simulink model "sampleModel1760"  (R2023a)
settings: Solver=VariableStepAuto  StartTime=0.0  StopTime=10.0  RelTol=1e-3
libraries: hdlsllib x6, simulink x5
settings Model: Creator=user1  LastModifiedBy=user1

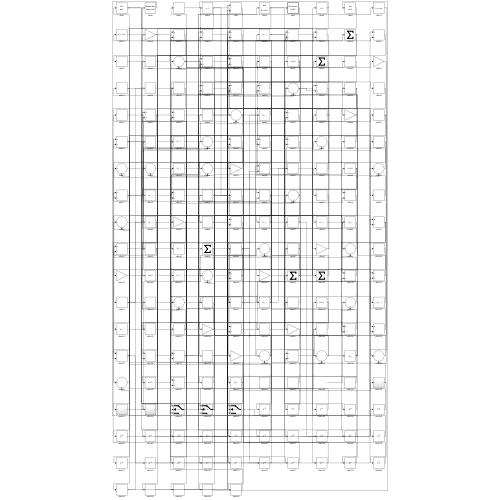
[thumbnail: Simulink's stored preview of the top-level diagram]
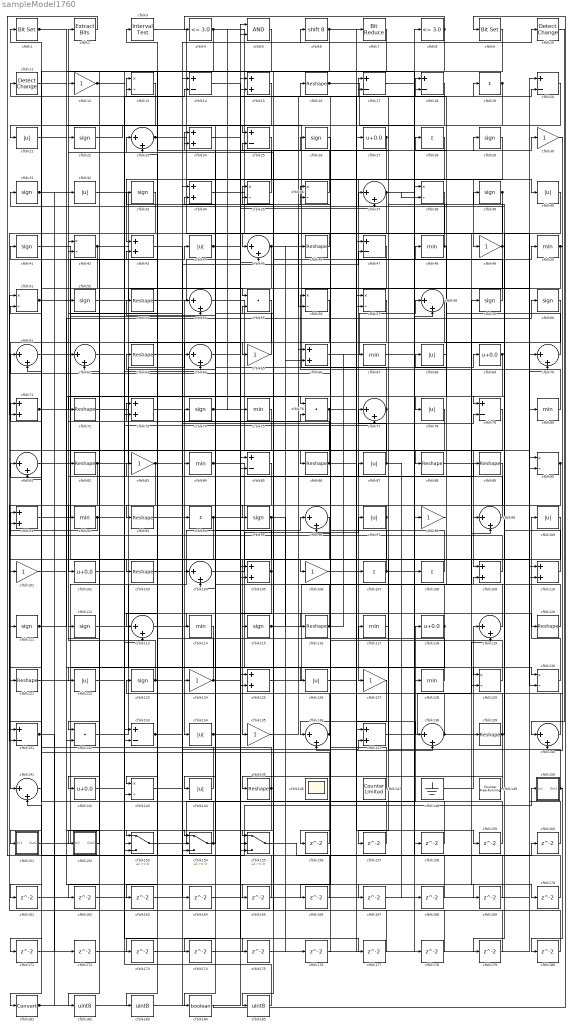
== system sampleModel1760 ==
  cfblk1 : simulink/Logic and Bit Operations/Bit Set  iBit=0
      settings: LibrarySourceBlock=|
      | hdlsllib/Logic and Bit
      | Operations/Bit Set
  cfblk10 : simulink/Logic and Bit Operations/Detect Change  vinit=0  OutDataTypeStr=boolean
      settings: LibrarySourceBlock=|
      | hdlsllib/Logic and Bit
      | Operations/Detect
      | Change
  cfblk{21,32,40,44,68,78,87,97,100,122,126,134,144} (13 alike) : Abs  SaturateOnIntegerOverflow=off
  cfblk{12,30,49,65,83,98,101,106,124,127,135} (11 alike) : Gain
  cfblk{27,69,102,118,142} (5 alike) : Bias  Bias=0.0  SaturateOnIntegerOverflow=off
  cfblk{16,46,53,63,72,82,86,88..89,93,103,116,120..121,139,145} (16 alike) : Reshape
  cfblk{23,37,45,54,58,61..62,64,70,77,81,96,99,104,113,119,136,138,140..141} (20 alike) : Sum  Inputs=|++
  cfblk{15,24,34,43,66,71,73,91,105,109..110,125,137} (13 alike) : Sum
  cfblk{19,28,94,107..108} (5 alike) : Sum  Inputs=+
  cfblk11 : simulink/Logic and Bit Operations/Detect Change  vinit=0  OutDataTypeStr=boolean
      settings: LibrarySourceBlock=|
      | hdlsllib/Logic and Bit
      | Operations/Detect
      | Change
  cfblk{22,26,29,31,33,39,41,52,59..60,74,95,111..112,115,123} (16 alike) : Signum
  cfblk{48,50,67,75,80,84,92,114,117,128} (10 alike) : MinMax
  cfblk{13,35..36,38,42,51,56..57,90,129..130,143} (12 alike) : Product  Inputs=*/  RndMeth=Zero  SaturateOnIntegerOverflow=on
  cfblk{14,17..18,20,25,47,79,85,131,133} (10 alike) : Sum  Inputs=+-
  cfblk132 : DotProduct  OutDataTypeStr=Inherit: Inherit via internal rule
  cfblk146 : Scope
      settings: Floating=on
  cfblk147 : hdlsllib/Sources/Counter Limited  uplimit=7  tsamp=-1
  cfblk148 : Ground
  cfblk149 : hdlsllib/Sources/Counter Free-Running  NumBits=16  tsamp=-1
  cfblk150 : Subsystem
      settings: LibrarySourceBlock=|
      | hdlsllib/Ports &
      | Subsystems/Subsystem
  cfblk151 : Subsystem
      settings: LibrarySourceBlock=|
      | hdlsllib/Ports &
      | Subsystems/Subsystem
  cfblk152 : Subsystem
      settings: LibrarySourceBlock=|
      | hdlsllib/Ports &
      | Subsystems/Subsystem
  cfblk153 : Switch  SaturateOnIntegerOverflow=off  InputSameDT=off
  cfblk154 : Switch  SaturateOnIntegerOverflow=off  InputSameDT=off
  cfblk155 : Switch  SaturateOnIntegerOverflow=off  InputSameDT=off
  cfblk{156..180} (25 alike) : Delay  SampleTime=1
  cfblk181 : DataTypeConversion  SaturateOnIntegerOverflow=off  RndMeth=Floor
  cfblk182 : DataTypeConversion  OutDataTypeStr=uint8  SaturateOnIntegerOverflow=off  RndMeth=Floor
  cfblk183 : DataTypeConversion  OutDataTypeStr=uint8  SaturateOnIntegerOverflow=off  RndMeth=Floor
  cfblk184 : DataTypeConversion  OutDataTypeStr=boolean  SaturateOnIntegerOverflow=off  RndMeth=Floor
  cfblk185 : DataTypeConversion  OutDataTypeStr=uint8  SaturateOnIntegerOverflow=off  RndMeth=Floor
  cfblk2 : simulink/Logic and Bit Operations/Extract Bits  bitsToExtract=Upper half  numBits=8  bitIdxRange=[0 7]  outScalingMode=Preserve fixed-point scaling
      settings: LibrarySourceBlock=|
      | hdlsllib/Logic and Bit
      | Operations/Extract Bits
  cfblk3 : hdlsllib/Logic and Bit Operations/Interval Test  IntervalClosedRight=on  uplimit=0.5  IntervalClosedLeft=on  lowlimit=-0.5  OutDataTypeStr=boolean
  cfblk4 : hdlsllib/Logic and Bit Operations/Compare To Constant  relop=<=  const=3.0  OutDataTypeStr=boolean
  cfblk5 : Logic  AllPortsSameDT=off  OutDataTypeStr=boolean
  cfblk55 : DotProduct  OutDataTypeStr=Inherit: Inherit via internal rule
  cfblk6 : ArithShift  BitShiftNumber=8
  cfblk7 : hdlsllib/Logic and Bit Operations/Bit Reduce  mode=AND
  cfblk76 : DotProduct  OutDataTypeStr=Inherit: Inherit via internal rule
  cfblk8 : hdlsllib/Logic and Bit Operations/Compare To Constant  relop=<=  const=3.0  OutDataTypeStr=boolean
  cfblk9 : simulink/Logic and Bit Operations/Bit Set  iBit=0
      settings: LibrarySourceBlock=|
      | hdlsllib/Logic and Bit
      | Operations/Bit Set
  wires:
  cfblk95/1 -> cfblk135/1, cfblk66/2, cfblk176/1
  cfblk116/1 -> cfblk23/1, cfblk67/1, cfblk16/1
  cfblk130/1 -> cfblk100/1
  cfblk123/1 -> cfblk2/1, cfblk76/2
  cfblk70/1 -> cfblk12/1
  cfblk85/1 -> cfblk102/1
  cfblk81/1 -> cfblk44/1
  cfblk66/1 -> cfblk58/1
  cfblk22/1 -> cfblk69/1
  cfblk58/1 -> cfblk106/1
  cfblk96/1 -> cfblk141/1
  cfblk46/1 -> cfblk45/1
  cfblk120/1 -> cfblk48/1
  cfblk114/1 -> cfblk143/1
  cfblk68/1 -> cfblk28/1
  cfblk110/1 -> cfblk31/1
  cfblk30/1 -> cfblk118/1
  cfblk53/1 -> cfblk30/1
  cfblk131/1 -> cfblk171/1, cfblk172/1
  cfblk34/1 -> cfblk58/2
  cfblk27/1 -> cfblk127/1, cfblk65/1
  cfblk44/1 -> cfblk88/1, cfblk17/2
  cfblk10/1 -> cfblk140/1
  cfblk80/1 -> cfblk56/1
  cfblk98/1 -> cfblk68/1
  cfblk55/1 -> cfblk134/1
  cfblk69/1 -> cfblk144/1, cfblk72/1
  cfblk26/1 -> cfblk86/1
  cfblk40/1 -> cfblk79/1
  cfblk59/1 -> cfblk22/1
  cfblk138/1 -> cfblk24/1, cfblk83/1, cfblk170/1
  cfblk93/1 -> cfblk94/1
  cfblk6/1 -> cfblk7/1, cfblk21/1, cfblk138/1
  cfblk153/1 -> cfblk128/1
  cfblk87/1 -> cfblk77/1, cfblk168/1
  cfblk117/1 -> cfblk37/1
  cfblk151/1(Out1) -> cfblk66/1
  cfblk107/1 -> cfblk8/1, cfblk61/1
  cfblk121/1 -> cfblk124/1
  cfblk143/1 -> cfblk36/1
  cfblk147/1 -> cfblk13/1
  cfblk125/1 -> cfblk27/1
  cfblk148/1 -> cfblk119/1
  cfblk5/1 -> cfblk181/1
  cfblk88/1 -> cfblk109/1
  cfblk51/1 -> cfblk84/1, cfblk154/2
  cfblk99/1 -> cfblk42/1
  cfblk128/1 -> cfblk41/1
  cfblk129/1 -> cfblk26/1
  cfblk57/1 -> cfblk111/1
  cfblk16/1 -> cfblk108/1, cfblk138/2
  cfblk84/1 -> cfblk129/1, cfblk29/1
  cfblk4/1 -> cfblk110/1, cfblk153/3, cfblk75/1
  cfblk83/1 -> cfblk79/2, cfblk143/2
  cfblk32/1 -> cfblk130/1
  cfblk134/1 -> cfblk96/1, cfblk37/2
  cfblk2/1 -> cfblk150/1(In1)
  cfblk74/1 -> cfblk15/1, cfblk99/2, cfblk177/1
  cfblk41/1 -> cfblk103/1
  cfblk18/1 -> cfblk131/1
  cfblk79/1 -> cfblk101/1
  cfblk124/1 -> cfblk52/1, cfblk89/1
  cfblk118/1 -> cfblk63/1, cfblk132/2, cfblk166/1
  cfblk11/1 -> cfblk154/1
  cfblk108/1 -> cfblk36/2
  cfblk48/1 -> cfblk78/1, cfblk13/2
  cfblk3/1 -> cfblk139/1
  cfblk36/1 -> cfblk3/1
  cfblk150/1(Out1) -> cfblk117/1, cfblk180/1
  cfblk140/1 -> cfblk87/1
  cfblk21/1 -> cfblk153/1
  cfblk126/1 -> cfblk107/1
  cfblk45/1 -> cfblk80/1, cfblk73/2
  cfblk12/1 -> cfblk105/2, cfblk162/1
  cfblk52/1 -> cfblk55/1
  cfblk25/1 -> cfblk43/1
  cfblk43/1 -> cfblk120/1
  cfblk7/1 -> cfblk142/1
  cfblk78/1 -> cfblk121/1
  cfblk119/1 -> cfblk17/1
  cfblk133/1 -> cfblk137/2, cfblk47/2
  cfblk115/1 -> cfblk59/1, cfblk46/1
  cfblk38/1 -> cfblk57/2
  cfblk152/1(Out1) -> cfblk112/1
  cfblk111/1 -> cfblk60/1, cfblk82/1
  cfblk104/1 -> cfblk97/1
  cfblk82/1 -> cfblk131/2, cfblk10/1
  cfblk60/1 -> cfblk93/1
  cfblk1/1 -> cfblk25/1, cfblk18/2
  cfblk132/1 -> cfblk14/1
  cfblk47/1 -> cfblk85/2
  cfblk105/1 -> cfblk74/1, cfblk155/3
  cfblk8/1 -> cfblk4/1, cfblk163/1
  cfblk65/1 -> cfblk33/1
  cfblk72/1 -> cfblk54/1
  cfblk112/1 -> cfblk126/1
  cfblk136/1 -> cfblk123/1, cfblk73/1
  cfblk94/1 -> cfblk130/2, cfblk133/2
  cfblk89/1 -> cfblk129/2
  cfblk15/1 -> cfblk152/1(In1)
  cfblk23/1 -> cfblk70/2, cfblk49/1
  cfblk35/1 -> cfblk11/1
  cfblk20/1 -> cfblk125/2
  cfblk149/1 -> cfblk145/1
  cfblk39/1 -> cfblk56/2, cfblk173/1
  cfblk91/1 -> cfblk34/1
  cfblk86/1 -> cfblk20/2, cfblk62/1
  cfblk49/1 -> cfblk132/1, cfblk24/2
  cfblk90/1 -> cfblk113/1, cfblk179/1
  cfblk76/1 -> cfblk50/1, cfblk104/1
  cfblk19/1 -> cfblk62/2, cfblk174/1
  cfblk127/1 -> cfblk136/1
  cfblk139/1 -> cfblk155/1, cfblk34/2, cfblk109/2, cfblk39/1
  cfblk102/1 -> cfblk115/1
  cfblk135/1 -> cfblk19/1
  cfblk145/1 -> cfblk42/2, cfblk154/3
  cfblk29/1 -> cfblk64/1
  cfblk42/1 -> cfblk155/2, cfblk151/1(In1)
  cfblk24/1 -> cfblk18/1
  cfblk122/1 -> cfblk77/2
  cfblk54/1 -> cfblk99/1
  cfblk14/1 -> cfblk40/1
  cfblk141/1 -> cfblk51/2
  cfblk77/1 -> cfblk53/1, cfblk184/1
  cfblk97/1 -> cfblk122/1, cfblk95/1
  cfblk154/1 -> cfblk71/1, cfblk104/2
  cfblk113/1 -> cfblk116/1
  cfblk71/1 -> cfblk54/2, cfblk90/2
  cfblk33/1 -> cfblk71/2
  cfblk144/1 -> cfblk81/1
  cfblk61/1 -> cfblk6/1
  cfblk142/1 -> cfblk64/2
  cfblk137/1 -> cfblk119/2
  cfblk37/1 -> cfblk98/1, cfblk38/2, cfblk92/1
  cfblk109/1 -> cfblk91/1
  cfblk73/1 -> cfblk35/1
  cfblk50/1 -> cfblk140/2, cfblk61/2
  cfblk92/1 -> cfblk14/2, cfblk91/2
  cfblk31/1 -> cfblk81/2, cfblk76/1
  cfblk28/1 -> cfblk156/1
  cfblk156/1 -> cfblk1/1
  cfblk100/1 -> cfblk157/1
  cfblk157/1 -> cfblk43/2
  cfblk17/1 -> cfblk158/1
  cfblk158/1 -> cfblk137/1
  cfblk106/1 -> cfblk159/1
  cfblk159/1 -> cfblk96/2
  cfblk155/1 -> cfblk160/1
  cfblk160/1 -> cfblk20/1
  cfblk56/1 -> cfblk161/1
  cfblk161/1 -> cfblk85/1
  cfblk162/1 -> cfblk57/1
  cfblk163/1 -> cfblk105/1
  cfblk63/1 -> cfblk164/1
  cfblk164/1 -> cfblk70/1
  cfblk101/1 -> cfblk165/1
  cfblk165/1 -> cfblk141/2
  cfblk166/1 -> cfblk35/2
  cfblk103/1 -> cfblk167/1
  cfblk167/1 -> cfblk110/2
  cfblk168/1 -> cfblk38/1
  cfblk64/1 -> cfblk169/1
  cfblk169/1 -> cfblk125/1
  cfblk170/1 -> cfblk23/2
  cfblk171/1 -> cfblk45/2
  cfblk172/1 -> cfblk113/2
  cfblk173/1 -> cfblk47/1
  cfblk174/1 -> cfblk15/2
  cfblk62/1 -> cfblk175/1
  cfblk175/1 -> cfblk90/1
  cfblk176/1 -> cfblk136/2
  cfblk177/1 -> cfblk133/1
  cfblk67/1 -> cfblk178/1
  cfblk178/1 -> cfblk51/1
  cfblk179/1 -> cfblk25/2
  cfblk180/1 -> cfblk55/2
  cfblk181/1 -> cfblk114/1, cfblk32/1
  cfblk13/1 -> cfblk182/1
  cfblk182/1 -> cfblk5/1
  cfblk75/1 -> cfblk183/1
  cfblk183/1 -> cfblk5/2
  cfblk184/1 -> cfblk9/1
  cfblk9/1 -> cfblk185/1
  cfblk185/1 -> cfblk153/2

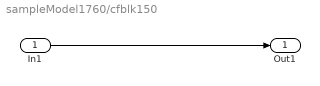
== system sampleModel1760/cfblk150 ==
  In1 : Inport
  Out1 : Outport
  wires:
  In1/1 -> Out1/1

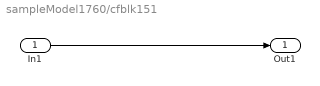
== system sampleModel1760/cfblk151 ==
  In1 : Inport
  Out1 : Outport
  wires:
  In1/1 -> Out1/1

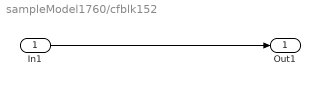
== system sampleModel1760/cfblk152 ==
  In1 : Inport
  Out1 : Outport
  wires:
  In1/1 -> Out1/1
